simulink subsystem "AVE_TEMPLATE_MESSAGE_PACK"  (R2024a)
settings: Solver=VariableStepAuto  StartTime=0.0  StopTime=10.0  RelTol=1e-3
libraries: etargetslib x1
settings Model: Creator=damerius  LastModifiedBy=Scythe
settings SolverCC: AlgebraicLoopSolver=TrustRegion
settings OptimizationCC: ReuseModelBlockBuffer=off
settings DebuggingCC: UnconnectedInputMsg=warning  UnconnectedOutputMsg=warning  UnconnectedLineMsg=warning
settings ModelReferenceCC: EnableRefExpFcnMdlSchedulingChecks=on
settings RTWCC: GPUComputeCapability=3.5  DLArmComputeVersion=19.05

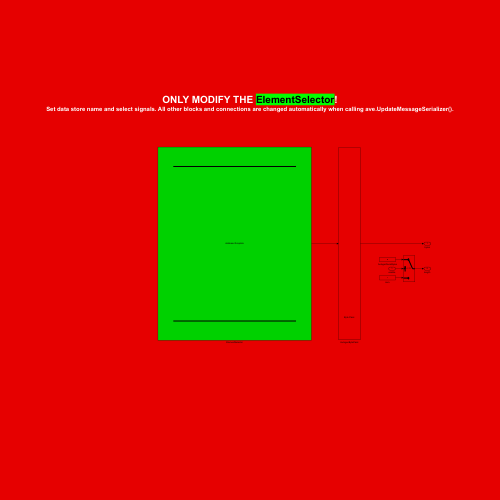
[thumbnail: Simulink's stored preview of the top-level diagram]
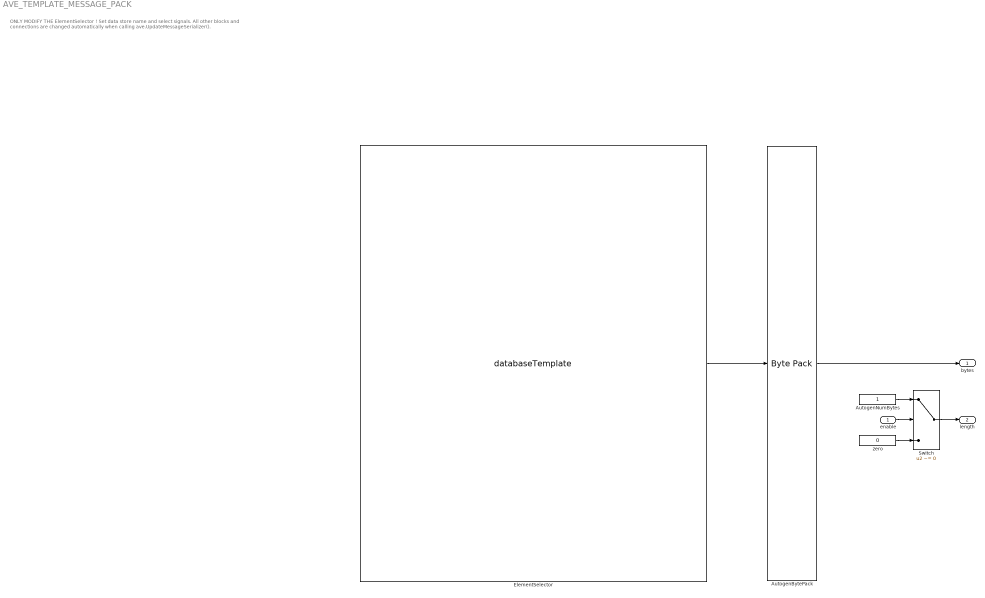
== system AVE_TEMPLATE_MESSAGE_PACK ==
  note: ONLY MODIFY THE ElementSelector !
      | Set data store name and select signals. All other blocks and connections are changed automatically when calling ave.UpdateMessageSerializer().
  enable : Inport  OutDataTypeStr=boolean  PortDimensions=1
  AutogenBytePack : etargetslib/Byte Pack  datatypes={'uint8'}  byteAlign=1
  AutogenNumBytes : Constant  OutDataTypeStr=uint32
  ElementSelector : DataStoreRead  DataStoreName=databaseTemplate  IndexOptions=Index vector (dialog)  Indices=1  OutputSizes=1
  Switch : Switch  Criteria=u2 ~= 0  SaturateOnIntegerOverflow=off  InputSameDT=off
  zero : Constant  Value=0  OutDataTypeStr=uint32
  bytes : Outport  OutDataTypeStr=uint8
  length : Outport  Port=2  OutDataTypeStr=uint32  PortDimensions=1
  wires:
  AutogenNumBytes/1 -> Switch/1
  AutogenBytePack/1 -> bytes/1
  enable/1 -> Switch/2
  zero/1 -> Switch/3
  Switch/1 -> length/1
  ElementSelector/1 -> AutogenBytePack/1
